simulink model "model_4_exact"  (R2021b)
settings: Solver=VariableStepAuto  StartTime=0.0  StopTime=2e8
values from neighbouring files (symbols this model uses):
  params = 0    [Combo_OT.m]
undefined symbols (not defined in the file or in its folder): mp_0, mp_f
settings Model: Creator=Mehdi  LastModifiedBy=Mehdi

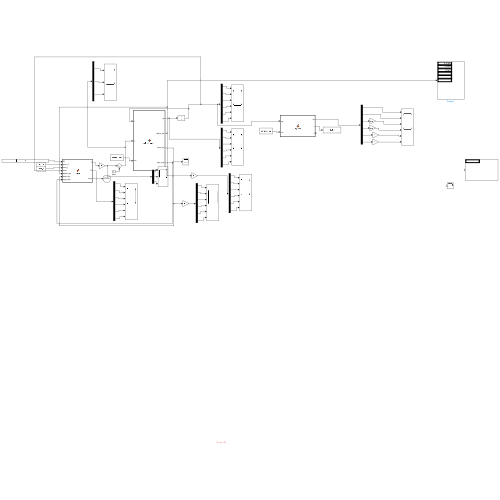
[thumbnail: Simulink's stored preview of the top-level diagram]
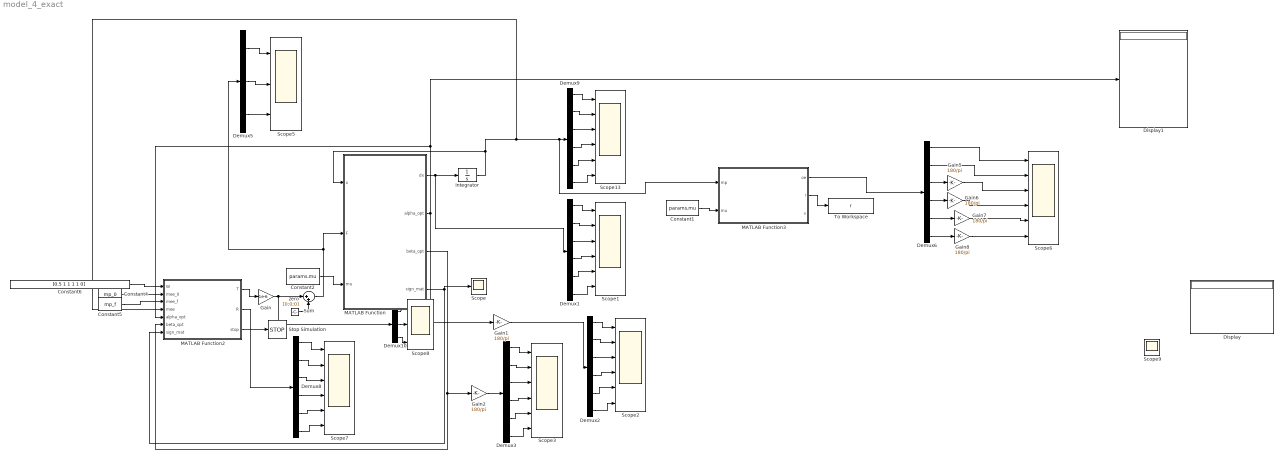
== system model_4_exact ==
  Constant1 : Constant  Value=params.mu
  Constant2 : Constant  Value=params.mu
  Constant4 : Constant  Value=mp_0
  Constant5 : Constant  Value=mp_f
  Constant6 : Constant  Value=[0.5 1 1 1 1 0]
  Demux{1..3,6,8..9} (6 alike) : Demux  Outputs=6
  Demux10 : Demux  Outputs=3
  Demux5 : Demux  Outputs=3
  Display : Display
  Display1 : Display
  Gain : Gain  Gain=1e-6
  Gain{1..2,5..8} (6 alike) : Gain  Gain=180/pi
  Integrator : Integrator  InitialCondition=mp_0
  MATLAB Function : MATLAB Function  TreatAsAtomicUnit=on
  MATLAB Function2 : MATLAB Function  TreatAsAtomicUnit=on
  MATLAB Function3 : MATLAB Function  TreatAsAtomicUnit=on
  Scope : Scope
  Scope{1..3,6..7,13} (6 alike) : Scope  NumInputPorts=6
  Scope5 : Scope  NumInputPorts=3
  Scope8 : Scope  NumInputPorts=3
  Scope9 : Scope
  Stop Simulation : Stop
  Sum : Sum  Inputs=|++
  To Workspace : ToWorkspace  VariableName=r  SaveFormat=Timeseries  SampleTime=-1
  zero : Constant  Value=[0;0;0]
  wires:
  Integrator/1 -> MATLAB Function2/4(mee), MATLAB Function3/1(mp), Demux9/1, MATLAB Function/1(x)
  Constant2/1 -> MATLAB Function/3(mu)
  Demux9/5 -> Scope13/5
  Demux9/1 -> Scope13/1
  Demux9/4 -> Scope13/4
  Demux9/3 -> Scope13/3
  Demux9/2 -> Scope13/2
  Demux9/6 -> Scope13/6
  Demux1/6 -> Scope1/6
  Demux1/2 -> Scope1/2
  Demux1/3 -> Scope1/3
  Demux1/4 -> Scope1/4
  Demux1/1 -> Scope1/1
  Demux1/5 -> Scope1/5
  Demux2/6 -> Scope2/6
  Demux2/2 -> Scope2/2
  Demux2/3 -> Scope2/3
  Demux2/4 -> Scope2/4
  Demux2/1 -> Scope2/1
  Demux2/5 -> Scope2/5
  MATLAB Function/2(alpha_opt) -> Display1/1, MATLAB Function2/5(alpha_opt), Gain1/1
  MATLAB Function/3(beta_opt) -> MATLAB Function2/6(beta_opt), Gain2/1
  Demux3/5 -> Scope3/5
  Demux3/1 -> Scope3/1
  Demux3/4 -> Scope3/4
  Demux3/3 -> Scope3/3
  Demux3/2 -> Scope3/2
  Demux3/6 -> Scope3/6
  Constant4/1 -> MATLAB Function2/2(mee_0)
  Constant5/1 -> MATLAB Function2/3(mee_f)
  Constant6/1 -> MATLAB Function2/1(W)
  Demux5/3 -> Scope5/3
  Demux5/2 -> Scope5/2
  Demux5/1 -> Scope5/1
  MATLAB Function2/1(T) -> Gain/1
  zero/1 -> Sum/2
  Gain/1 -> Sum/1, Demux10/1
  MATLAB Function2/3(stop) -> Stop Simulation/1
  Demux6/6 -> Gain8/1
  Demux6/3 -> Gain5/1
  Demux6/4 -> Gain6/1
  Demux6/5 -> Gain7/1
  MATLAB Function3/1(oe) -> Demux6/1
  Demux8/4 -> Scope7/4
  Demux8/3 -> Scope7/3
  Demux8/5 -> Scope7/5
  Demux8/2 -> Scope7/2
  Demux8/6 -> Scope7/6
  Demux8/1 -> Scope7/1
  MATLAB Function2/2(R) -> Demux8/1
  Gain1/1 -> Demux2/1
  MATLAB Function/1(dx) -> Demux1/1, Integrator/1
  Gain2/1 -> Demux3/1
  Demux6/1 -> Scope6/1
  Demux6/2 -> Scope6/2
  Gain5/1 -> Scope6/3
  Gain6/1 -> Scope6/4
  Gain7/1 -> Scope6/5
  Gain8/1 -> Scope6/6
  Demux10/2 -> Scope8/2
  Demux10/1 -> Scope8/1
  Demux10/3 -> Scope8/3
  ? -> ?
  Sum/1 -> MATLAB Function/2(F), Demux5/1
  MATLAB Function/4(sign_mat) -> Scope/1, MATLAB Function2/7(sign_mat)
  Constant1/1 -> MATLAB Function3/2(mu)
  MATLAB Function3/2(r) -> To Workspace/1

== matlab function model_4_exact/MATLAB Function ==
  data: x input; F input; dx output; mu input; alpha_opt output; beta_opt output; sign_mat output
function [dx,alpha_opt,beta_opt,sign_mat] = path_dynamics(x,F,mu)


%%%% to be optimized

% a
% ep1=e*sin(omega+OMEGA);
% ep2=e*cos(omega+OMEGA);
% zig1=tan(inc/2)*sin(OMEGA);
% zig2=tan(inc/2)*cos(OMEGA);
% lambda=theta+omega+OMEGA;


a=x(1);
ep1=x(2);
ep2=x(3);
zig1=x(4);
zig2=x(5);
lambda=x(6);

slam=sin(lambda);
clam=cos(lambda);
L=a*(1-ep1^2-ep2^2);
h=sqrt(mu*L);
r=L/(1+ep1*slam+ep2*clam);

%%% to be optimized!



a_dot_=2*a^2/h*[ep2*slam-ep1*clam L/r 0];
ep1_dot_=r/h*[-L/r*clam ep1+(1+L/r)*slam -ep2*(zig1*clam-zig2*slam)];
ep2_dot_=r/h*[L/r*slam ep2+(1+L/r)*clam ep1*(zig1*clam-zig2*slam)];
zig1_dot_=r/(2*h)*[0 0 (1+zig1^2+zig2^2)*slam];
zig2_dot_=r/(2*h)*[0 0 (1+zig1^2+zig2^2)*clam];
lambda_dot_=r/h*[0 0 zig2*slam-zig1*clam];


a_dot=dot(a_dot_,F);
ep1_dot=dot(ep1_dot_,F);
ep2_dot=dot(ep2_dot_,F);
zig1_dot=dot(zig1_dot_,F);
zig2_dot=dot(zig2_dot_,F);
lambda_dot=h/r^2+dot(lambda_dot_,F);

% % % a_dot=2*a^2/h*dot([ep2*slam-ep1*clam L/r 0],F);
% % % ep1_dot=r/h*dot([-L/r*clam ep1+(1+L/r)*slam -ep2*(zig1*clam-zig2*slam)],F);
% % % ep2_dot=r/h*dot([L/r*slam ep2+(1+L/r)*clam ep1*(zig1*clam-zig2*slam)],F);
% % % zig1_dot=r/(2*h)*dot([0 0 (1+zig1^2+zig2^2)*slam],F);
% % % zig2_dot=r/(2*h)*dot([0 0 (1+zig1^2+zig2^2)*clam],F);
% % % lambda_dot=h/r^2+r/h*dot([0 0 zig2*slam-zig1*clam],F);

% dx=zeros(6,1);

dx=[a_dot;ep1_dot;ep2_dot;zig1_dot;zig2_dot;lambda_dot];


% sign_mat=sign([ep2*slam-ep1*clam L/r 0;-L/r*clam ep1+(1+L/r)*slam -ep2*(zig1*clam-zig2*slam);L/r*slam ep2+(1+L/r)*clam ep1*(zig1*clam-zig2*slam);0 0 (1+zig1^2+zig2^2)*slam;0 0 (1+zig1^2+zig2^2)*clam;0 0 zig2*slam-zig1*clam]);
% sign_mat=sign([ep2*slam-ep1*clam 1 0;-clam ep1+(1+L/r)*slam -ep2*(zig1*clam-zig2*slam);slam ep2+(1+L/r)*clam ep1*(zig1*clam-zig2*slam);0 0 slam;0 0 clam;0 0 zig2*slam-zig1*clam]);



% [a e i omega OMEGA theta]

alpha_opt=zeros(6,1);
beta_opt=zeros(6,1);


%%% based on oe
% % % ep1plus=ep1*slam+ep2*clam;
% % % ep2minus=ep2*slam-ep2*clam;
% % % zig1c=zig1*clam-zig2*slam;
% % % zig2s=zig2*slam-zig1*clam;
% % % alpha_opt(1)=atan((r/L)*ep2minus);
% % % alpha_opt(2)=atan((L/r*ep2minus)/(ep1^2+ep2^2+(1+L/r)*ep1plus));
% % % beta_opt(3)=sign(zig1*slam+zig2*clam)*pi/2;
% % % beta_opt(4)=sign(zig2s)*pi/2;
% % % alpha_opt(5)=atan(-L/(L+r)*(ep1plus/ep2minus));
% % % sinaw=sin(alpha_opt(5));
% % % cosaw=cos(alpha_opt(5));
% % % beta_opt(5)=atan((-(ep1^2+ep2^2)/(zig1^2+zig2^2))*((r*(zig1^2+zig2^2)*zig2s+r/2*(1+zig1^2+zig2^2)*zig1c)/(L*ep1plus*sinaw-(L+r)*ep2minus*cosaw)));
% alpha_opt(6)=atan(-L/(L+r)*ep1plus/ep2minus);
% beta_opt(6)=


alpha_opt(1)=atan(r/L*(ep2*slam-ep1*clam));
alpha_opt(2)=atan(-L*clam/(r*ep1+(r+L)*slam));
alpha_opt(3)=atan(L*slam/(r*ep2+(r+L)*clam));


beta_opt(2)=atan(r*ep2*(zig1*clam-zig2*slam)/(L*clam*sin(alpha_opt(2))-(r*ep1+(r+L)*slam)*cos(alpha_opt(2))));
beta_opt(3)=atan(r*ep1*(zig1*clam-zig2*slam)/(L*slam*sin(alpha_opt(3))-(r*ep2+(r+L)*clam)*cos(alpha_opt(3))));

beta_opt(4)=sign(slam)*pi/2;
beta_opt(5)=sign(clam)*pi/2;

beta_opt(6)=sign(zig2*slam-zig1*clam)*pi/2;


% e=sqrt(ep1^2+ep2^2);
% inc=2*atan(sqrt(zig1^2+zig2^2));
% OMEGA=atan(zig1/zig2);
% omega=atan(ep1/ep2)-OMEGA;
% theta=lambda-atan(ep1/ep2);

% 
% F_sample=zeros(3,6);
% sign_vec=zeros(6,2);

% for i=1:6
%     F_sample(:,i)=[sin(alpha_opt(i))*cos(beta_opt(i));cos(alpha_opt(i))*cos(beta_opt(i));sin(beta_opt(i))];
% end

% for i=1:6
%     F_sample(:,i)=[sin(alpha_opt(i));cos(alpha_opt(i));0];
% end
% 
% sign_vec(1,1)=2*a^2/h*dot([ep2*slam-ep1*clam L/r 0],F_sample(:,1));
% sign_vec(2,1)=r/h*dot([-L/r*clam ep1+(1+L/r)*slam -ep2*(zig1*clam-zig2*slam)],F_sample(:,2));
% sign_vec(3,1)=r/h*dot([L/r*slam ep2+(1+L/r)*clam ep1*(zig1*clam-zig2*slam)],F_sample(:,3));
% sign_vec(4,1)=r/(2*h)*dot([0 0 (1+zig1^2+zig2^2)*slam],F_sample(:,4));
% sign_vec(5,1)=r/(2*h)*dot([0 0 (1+zig1^2+zig2^2)*clam],F_sample(:,5));
% sign_vec(6,1)=h/r^2+r/h*dot([0 0 zig2*slam-zig1*clam],F_sample(:,6));
% 
% for i=1:6
%     F_sample(:,i)=[0;cos(beta_opt(i));sin(beta_opt(i))];
% end
% 
% 
% 
% sign_vec(1,2)=2*a^2/h*dot([ep2*slam-ep1*clam L/r 0],F_sample(:,1));
% sign_vec(2,2)=r/h*dot([-L/r*clam ep1+(1+L/r)*slam -ep2*(zig1*clam-zig2*slam)],F_sample(:,2));
% sign_vec(3,2)=r/h*dot([L/r*slam ep2+(1+L/r)*clam ep1*(zig1*clam-zig2*slam)],F_sample(:,3));
% sign_vec(4,2)=r/(2*h)*dot([0 0 (1+zig1^2+zig2^2)*slam],F_sample(:,4));
% sign_vec(5,2)=r/(2*h)*dot([0 0 (1+zig1^2+zig2^2)*clam],F_sample(:,5));
% sign_vec(6,2)=h/r^2+r/h*dot([0 0 zig2*slam-zig1*clam],F_sample(:,6));
% 
% sign_vec=sign(sign_vec);





% sign_mat=zeros(6,3);
% 
% sign_mat(1,:)=[ep2*slam-ep1*clam L/r 0];
% sign_mat(2,:)=[-L/r*clam ep1+(1+L/r)*slam -ep2*(zig1*clam-zig2*slam)];
% sign_mat(3,:)=[L/r*slam ep2+(1+L/r)*clam ep1*(zig1*clam-zig2*slam)];
% sign_mat(4,:)=[0 0 (1+zig1^2+zig2^2)*slam];
% sign_mat(5,:)=[0 0 (1+zig1^2+zig2^2)*clam];
% sign_mat(6,:)=[0 0 zig2*slam-zig1*clam];
% 
% sign_mat=sign(sign_mat);


sign_mat=sign([a_dot_;ep1_dot_;ep2_dot_;zig1_dot_;zig2_dot_;lambda_dot_]);




end

== matlab function model_4_exact/MATLAB Function2 ==
  data: W input; mee_0 input; mee_f input; mee input; alpha_opt input; beta_opt input; T output; R output; stop output; sign_mat input
function [T,R,stop]  = Guider(W,mee_0,mee_f,mee,alpha_opt,beta_opt,sign_mat)


stop=0;

% mark=0;

R=zeros(6,1);
ss=ones(6,1);

%
% ss(1)=-1;
% ss(2)=-1;
% % ss(4)=-1;

T=[0;0;0];

% for i=1:5
%
%     %     if abs(mee_f(i)-mee_0(i))>1e-5 && abs(mee_f(i)-mee(i))>1e-5
%
%     if abs(mee_f(i)-mee_0(i))>1e-5
%
%         R(i)=abs((mee(i)-mee_f(i))/(mee_f(i)-mee_0(i)));
%
%         %         if  abs(R(i))>5
%         %             R(i)=5;
%         %         end
%         %         if  abs(R(i))<-5
%         %             R(i)=-5;
%         %         end
%
%     else
%         R(i)=0;
%     end
% end


for i=1:6

    %     if abs(mee_f(i)-mee_0(i))>1e-5 && abs(mee_f(i)-mee(i))>1e-5
    %      ss(i)=sign(oe_f(i)-oe(i));

    if abs(mee_f(i)-mee_0(i))>1e-5

        R(i)=abs((mee_f(i)-mee(i))/(mee_f(i)-mee_0(i)));

        %         if  abs(R(i))>5
        %             R(i)=5;
        %         end
        %         if  abs(R(i))<-5
        %             R(i)=-5;
        %         end


    else
        R(i)=0;
    end
end



if norm(R)<1e-2
    stop=1;
end

% ss(1)=-1;

% alpha_opt1=zeros(6,1);
% beta_opt1=zeros(6,1);


alpha_opt1=alpha_opt;
beta_opt1=beta_opt;



% % % ss(1)=sign(mee_f(1)-mee(1));  %% sign ok
% % % ss(2)=-sign(mee_f(2)-mee(2));  %% sign ok
% % % ss(3)=-sign(mee_f(3)-mee(3));
% % % ss(4)=sign(mee_f(4)-mee(4));
% % % ss(5)=sign(mee_f(5)-mee(5));
% % % ss(6)=sign(mee_f(6)-mee(6));

% ss=R_dot;

% ang1=rem(x(6)+2*pi,2*pi);
% if ang1>pi
%     ss(2)=-ss(2);
% alpha_opt(2)=2*pi-alpha_opt(2);
% end

% n=0;

%
% if mee_f(1)<mee(1)
%     ss(1)=-1;
% end
%
% if mee_f(2)<mee(2)
%     ss(2)=-1;
% end

% sign_mat1=ones(6,3);

% for i=1:6
%     for j=1:3
%         if (sign_mat(i,j)<0 && mee_f(i)>mee(i)) || (sign_mat(i,j)>0 && mee_f(i)<mee(i))
%             sign_mat1(i,j)=-1;
%         end
%     end
%
% end

% for i=1:6
%         if (sign_vec(i,1)<0 && mee_f(i)>mee(i)) || (sign_vec(i,1)>0 && mee_f(i)<mee(i)) || (sign_vec(i,2)<0 && mee_f(i)>mee(i)) || (sign_vec(i,2)>0 && mee_f(i)<mee(i))
%             ss(i)=-1;
%         end
% 
% end


% for i=1:6
%     if (sign_vec(i,1)<0 && oe_f(i)>oe(i)) || (sign_vec(i,1)>0 && oe_f(i)<oe(i))
%         alpha_opt1(i)= -alpha_opt(i);
%     end
% 
%     if (sign_vec(i,2)<0 && oe_f(i)>oe(i)) || (sign_vec(i,2)>0 && oe_f(i)<oe(i))
%         beta_opt1(i)= -beta_opt(i);
%     end
% end


% for i=1:6
%     if (sign_vec(i,1)<0 && R(i)>0) || (sign_vec(i,1)>0 && R(i)<0)
%         alpha_opt1(i)= -alpha_opt(i);
%     end
% 
%     if (sign_vec(i,2)<0 && R(i)>0) || (sign_vec(i,2)>0 && R(i)<0)
%         beta_opt1(i)= -beta_opt(i);
%     end
% end

% for i=1:5
%     if sign_vec(i,1)<0
%         alpha_opt1(i)= pi+alpha_opt(i);
%     end
% 
%     if sign_vec(i,2)<0
%         beta_opt1(i)= pi+beta_opt(i);
%     end
% end



% for i=1:5
%     s1=0;
%     s2=0;
%     if (sign_vec(i,1)==-1  && mee_f(i)>mee(i)) || (sign_vec(i,1)==1 && mee_f(i)<mee(i))
% %         ss(i)=-1;
%                 alpha_opt1(i)=-alpha_opt1(i);
%         s1=1;
% 
%     end
% 
%     if (sign_vec(i,2)==-1  && mee_f(i)>mee(i)) || (sign_vec(i,2)==1 && mee_f(i)<mee(i))
% %         ss(i)=-1;
%                 beta_opt1(i)=-beta_opt1(i);
%         s2=1;
%     end
% 
%     if s1~=s2
%         mark=1;
%     end
% 
%     %     if (sign_vec(i,2)==-1  && mee_f(i)>mee(i)) || (sign_vec(i,2)==1 && mee_f(i)<mee(i))
%     %         beta_opt1(i)=pi+beta_opt1(i);
%     %     end
% end


ss_rsw=ones(6,3);

for i=1:6
    for j=1:3
        if (sign_mat(i,j)<0 && mee_f(i)>mee(i)) || (sign_mat(i,j)>0 && mee_f(i)<mee(i))
            ss_rsw(i,j)=-1;
        end
    end
end

for i=1:6

    %     n=n+1;
    %     ss=1;
    %     ang1=rem(x(6)+2*pi,2*pi);
    %     if ang1<pi
    %         alpha_opt(i)=-alpha_opt(i);
    % ss=-1;
    %     end

    %         ss=sign(x(i)-mp_f(i));
    %     ss=1;
    %
    % ss=-1;

    %     if (sign_mat(i,1)==-1  && mee_f(i)>mee(i)) || (sign_mat(i,1)==1 && mee_f(i)<mee(i))
    %         alpha_opt(i)=-abs(alpha_opt(i));
    %     else
    %         alpha_opt(i)=abs(alpha_opt(i));
    %     end
    %
    %     if (sign_mat(i,3)==-1  && mee_f(i)>mee(i)) || (sign_mat(i,3)==1 && mee_f(i)<mee(i))
    %         beta_opt(i)=-abs(beta_opt(i));
    %     else
    %         beta_opt(i)=abs(beta_opt(i));
    %     end

    %     if (sign_mat(i,1)==-1  && mee_f(i)>mee(i)) || (sign_mat(i,1)==1 && mee_f(i)<mee(i))
    %                 alpha_opt1(i)=-alpha_opt(i);
    % %         ss(i)=-1;
    %     else
    %                 alpha_opt1(i)=abs(alpha_opt(i));
    %     end
    %
    %     if (sign_mat(i,3)==-1  && mee_f(i)>mee(i)) || (sign_mat(i,3)==1 && mee_f(i)<mee(i))
    %                 beta_opt1(i)=-beta_opt(i);
    %     else
    %                 beta_opt1(i)=abs(beta_opt(i));
    %     end






%     T=T+ss(i)*W(i)*R(i)*([sin(alpha_opt1(i))*cos(beta_opt1(i));cos(alpha_opt1(i))*cos(beta_opt1(i));sin(beta_opt1(i))]);

    T=T+ss(i)*W(i)*R(i)*([ss_rsw(i,1)*abs(sin(alpha_opt1(i))*cos(beta_opt1(i)));ss_rsw(i,2)*abs(cos(alpha_opt1(i))*cos(beta_opt1(i)));ss_rsw(i,3)*abs(sin(beta_opt1(i)))]);

    % T=T+ss(n)*W(n)*R(i)*([sin(alpha_opt(i))*cos(0);cos(alpha_opt(i))*cos(0);sin(beta_opt(i))]);
    %
end

% for i=1:6
%     n=n+1;
%     ss=1;
%     ang1=rem(x(6)+2*pi,2*pi);
%     if ang1<pi
%         alpha_opt(i)=-alpha_opt(i);
% ss=-1;
%     end

%         ss=sign(x(i)-mp_f(i));
%     ss=1;
%
% ss=-1;
%     T=T+ss(i)*W(i)*R(i)*([sin(alpha_opt(i))*cos(beta_opt(i));cos(alpha_opt(i))*cos(beta_opt(i));sin(beta_opt(i))]);
% T=T+ss(i)*W(n)*R(i)*([sin(0)*cos(beta_opt(i));cos(0)*cos(beta_opt(i));sin(beta_opt(i))]);
%
% end

% T=T./sum(W);


T=T./sum(W);


% if norm(T)>1e-10
% 
%     T=T./norm(T);
% 
% else
%     T=[0;0;0];
% end

end

== matlab function model_4_exact/MATLAB Function3 ==
  data: mp input; oe output; mu input; r output; v output
function [oe,r,v]=mp2oe(mp,mu)





[r, v] = mee2rv(mp,mu);

oe = rv2oe (r, v,mu);




% % % % a=mp(1);
% % % % ep1=mp(2);
% % % % ep2=mp(3);
% % % % zig1=mp(4);
% % % % zig2=mp(5);
% % % % lambda=mp(6);
% % % % 
% % % % 
% % % % % % ep1=e*sin(omega+OMEGA);
% % % % % % ep2=e*cos(omega+OMEGA);
% % % % % % zig1=tan(inc/2)*sin(OMEGA);
% % % % % % zig2=tan(inc/2)*cos(OMEGA);
% % % % % % lambda=theta+omega+OMEGA;
% % % % % %
% % % % % % mp=[a;ep1;ep2;zig1;zig2;lambda];
% % % % 
% % % % %%% to be optimized
% % % % e=sqrt(ep1^2+ep2^2);
% % % % inc=2*atan(sqrt(zig1^2+zig2^2));
% % % % 
% % % % if inc==0
% % % %     OMEGA=0;
% % % % else
% % % %     tan1=tan(inc/2);
% % % %     OMEGA=atan3(zig1/tan1,zig2/tan1);
% % % % end
% % % % 
% % % % 
% % % % % if sign(zig2)*sign(cos(OMEGA))<0 || sign(zig1)*sign(sin(OMEGA))<0
% % % % %     inc=-inc;
% % % % % end
% % % % 
% % % % 
% % % % if OMEGA>pi
% % % %     OMEGA=OMEGA-2*pi;
% % % % end
% % % % 
% % % % % inc=inc*(sign(zig2)*sign(cos(OMEGA)));
% % % % 
% % % % if e==0
% % % %     omega=0;
% % % % else
% % % %     omega=atan3(ep1/e,ep2/e)-OMEGA;
% % % % end
% % % % 
% % % % if omega>2*pi
% % % %     omega=omega-2*pi;
% % % %     
% % % % end
% % % % 
% % % % 
% % % % theta=lambda-omega-OMEGA;
% % % % if theta<0
% % % %     theta=theta+2*pi;
% % % % end
% % % % 
% % % % if theta>2*pi
% % % %     theta=rem(theta,2*pi);
% % % % end
% % % % 
% % % % oe=[a;e;inc;omega;OMEGA;theta];


end
